simulink library "csc_valvesim_sim_lib"  (R2014b)
settings: Solver=ode45  StartTime=0.0  StopTime=10.0  RelTol=1e-3
libraries: util_info_lib x1, csu_mct_microcontroller_timer_sim_lib x1, csu_tss_thrustersim_sim_lib x1
settings Model: Creator=escrane  LastModifiedBy=mstewart

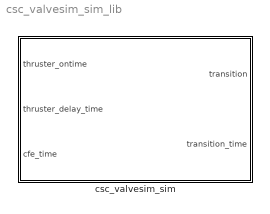
== system csc_valvesim_sim_lib ==
  csc_valvesim_sim : Subsystem  mask{thruster_idx=1, num_thrusters=26}
      mask prompts: thruster_idx "Index of Thruster (1-total)"; num_thrusters "Number of thrusters(total)"

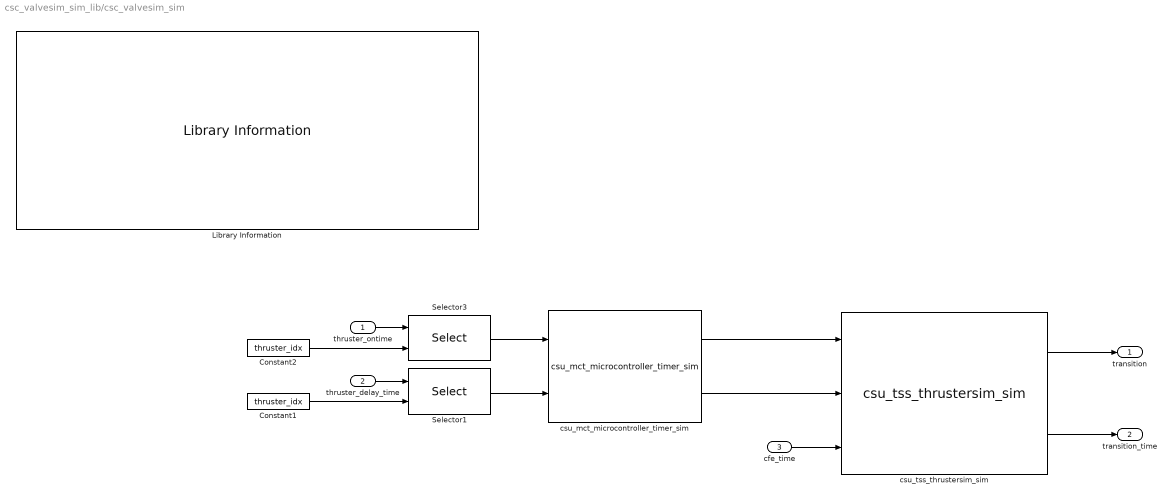
== system csc_valvesim_sim_lib/csc_valvesim_sim ==
  thruster_ontime : Inport
  thruster_delay_time : Inport  Port=2
  cfe_time : Inport  Port=3
  Constant1 : Constant  Value=thruster_idx  OutDataTypeStr=uint8
  Constant2 : Constant  Value=thruster_idx  OutDataTypeStr=uint8
  Library Information : util_info_lib/Library Information  owner='escrane'
  Selector1 : Selector  InputPortWidth=num_thrusters  IndexOptions=Index vector (port)  Indices=[1 3]
  Selector3 : Selector  InputPortWidth=num_thrusters  IndexOptions=Index vector (port)  Indices=[1 3]
  csu_mct_microcontroller_timer_sim : csu_mct_microcontroller_timer_sim_lib/csu_mct_microcontroller_timer_sim
  csu_tss_thrustersim_sim : csu_tss_thrustersim_sim_lib/csu_tss_thrustersim_sim
  transition : Outport
  transition_time : Outport  Port=2
  wires:
  Selector1/1 -> csu_mct_microcontroller_timer_sim/2
  thruster_delay_time/1 -> Selector1/1
  Constant1/1 -> Selector1/2
  thruster_ontime/1 -> Selector3/1
  csu_mct_microcontroller_timer_sim/1 -> csu_tss_thrustersim_sim/1
  csu_mct_microcontroller_timer_sim/2 -> csu_tss_thrustersim_sim/2
  cfe_time/1 -> csu_tss_thrustersim_sim/3
  Selector3/1 -> csu_mct_microcontroller_timer_sim/1
  Constant2/1 -> Selector3/2
  csu_tss_thrustersim_sim/1 -> transition/1
  csu_tss_thrustersim_sim/2 -> transition_time/1
